simulink model "PLANT_figura_9b"  (R2025b)
settings: Solver=VariableStepAuto  StartTime=0.0  StopTime=10.0  RelTol=1e-3
settings Model: Creator=super  LastModifiedBy=super

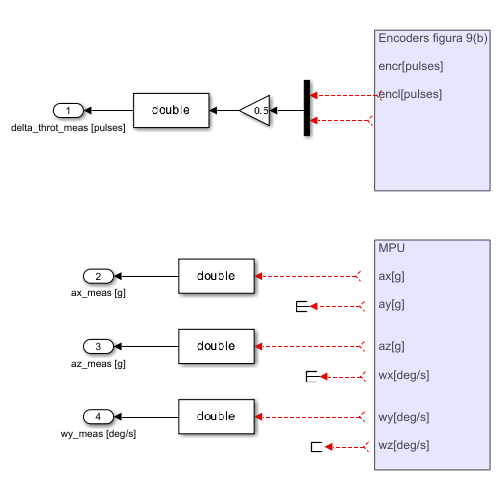
[thumbnail: Simulink's stored preview of the top-level diagram]
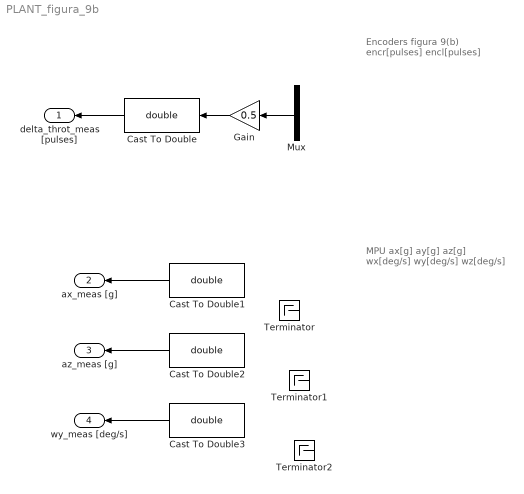
== system PLANT_figura_9b ==
  note: Encoders figura 9(b)
      |
      | encr[pulses]
      |
      | encl[pulses]
  note: MPU
      |
      | ax[g]
      |
      | ay[g]
      |
      |
      | az[g]
      |
      | wx[deg/s]
      |
      |
      | wy[deg/s]
      |
      | wz[deg/s]
  Cast To Double{,1..3} (4 alike) : DataTypeConversion  OutDataTypeStr=double  SaturateOnIntegerOverflow=off  RndMeth=Floor
  Gain : Gain  Gain=0.5
  Mux : Mux  Inputs=2
  Terminator : Terminator
  Terminator1 : Terminator
  Terminator2 : Terminator
  delta_throt_meas [pulses] : Outport
  ax_meas [g] : Outport  Port=2
  az_meas [g] : Outport  Port=3
  wy_meas [deg/s] : Outport  Port=4
  wires:
  Mux/1 -> Gain/1
  ? -> Mux/1
  ? -> Mux/2
  Gain/1 -> Cast To Double/1
  Cast To Double/1 -> delta_throt_meas [pulses]/1
  ? -> Cast To Double1/1
  ? -> Cast To Double2/1
  ? -> Cast To Double3/1
  Cast To Double1/1 -> ax_meas [g]/1
  Cast To Double2/1 -> az_meas [g]/1
  Cast To Double3/1 -> wy_meas [deg/s]/1
  ? -> Terminator/1
  ? -> Terminator1/1
  ? -> Terminator2/1
